simulink model "Test_Memory_Block_Word"  (Simulink 8.7)
settings: Solver=ode45  StartTime=0.0  StopTime=len  RelTol=1e-3
libraries: Miscellaneous x2, Memory_Blocks_Lib x1
settings Model: Creator=N  LastModifiedBy=Jozko Mrkvicka
settings DataIOCC: LimitDataPoints=off
settings DebuggingCC: UnderspecifiedInitializationDetection=Simplified  MergeDetectMultiDrivingBlocksExec=error
settings HardwareCC: ProdBitPerPointer=64  ProdLargestAtomicFloat=Float  ProdIntDivRoundTo=Zero  ProdEndianess=LittleEndian  ProdHWDeviceType=Intel->x86-64 (Windows64)
settings ModelReferenceCC: PropagateSignalLabelsOutOfModel=on

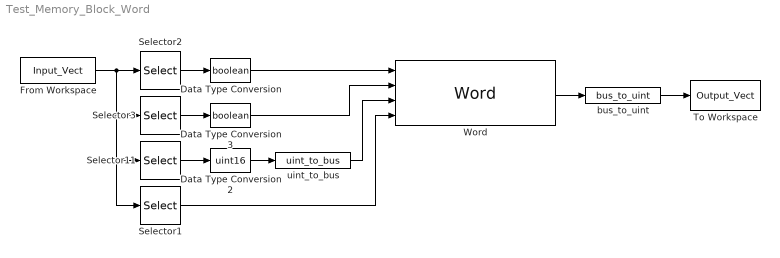
== system Test_Memory_Block_Word ==
  Data Type Conversion : DataTypeConversion  OutDataTypeStr=boolean
  Data Type Conversion2 : DataTypeConversion  OutDataTypeStr=uint16
  Data Type Conversion3 : DataTypeConversion  OutDataTypeStr=boolean
  From Workspace : FromWorkspace  VariableName=Input_Vect  SampleTime=1  Interpolate=off  OutputAfterFinalValue=Holding final value
  Selector1 : Selector  IndexMode=Zero-based  InputPortWidth=4  IndexOptions=Index vector (dialog)  Indices=3  OutputSizes=1
  Selector11 : Selector  IndexMode=Zero-based  InputPortWidth=4  IndexOptions=Index vector (dialog)  Indices=2  OutputSizes=1
  Selector2 : Selector  IndexMode=Zero-based  InputPortWidth=4  IndexOptions=Index vector (dialog)  Indices=0  OutputSizes=1
  Selector3 : Selector  IndexMode=Zero-based  InputPortWidth=4  IndexOptions=Index vector (dialog)  Indices=1  OutputSizes=1
  To Workspace : ToWorkspace  VariableName=Output_Vect  SampleTime=1
  Word : Memory_Blocks_Lib/Memory_Blocks_Lib/Word
  bus_to_uint : Miscellaneous/bus_to_uint
  uint_to_bus : Miscellaneous/uint_to_bus
  wires:
  Word/1 -> bus_to_uint/1
  bus_to_uint/1 -> To Workspace/1
  Selector11/1 -> Data Type Conversion2/1
  Selector2/1 -> Data Type Conversion/1
  Selector1/1 -> Word/4
  From Workspace/1 -> Selector3/1, Selector1/1, Selector11/1, Selector2/1
  Data Type Conversion/1 -> Word/1
  Data Type Conversion2/1 -> uint_to_bus/1
  Selector3/1 -> Data Type Conversion3/1
  Data Type Conversion3/1 -> Word/2
  uint_to_bus/1 -> Word/3
